simulink model "FourBarCrank_2"  (Simulink 7.0)
settings: Solver=ode1  StartTime=0.0  StopTime=inf  FixedStep=0.001  RelTol=1e-3
libraries: mblibv1 x23
settings Model: Creator=colinlea  LastModifiedBy=colinlea  ExtModeTrigDuration=10000
settings SolverCC: PositivePriorityOrder=on
settings RTWCC: SystemTargetFile=quarc_windows.tlc  TemplateMakefile=quarc_default_tmf  Description=QuaRC Win32 Target  ProcessScript=quarc_windows_make_rtw_hook
settings STFCustomTargetCC: TargetPreCompLibLocation=C:\DOCUME~1\ALLUSE~1\APPLIC~1\QuaRC\lib\2007b\windows\release  GenFloatMathFcnCalls=ANSI_C  SystemTargetFile=quarc_windows.tlc
settings GRTTargetCC: TargetPreCompLibLocation=C:\DOCUME~1\ALLUSE~1\APPLIC~1\QuaRC\lib\2007b\windows\release  CompOptLevelCompliant=off  MatFileLogging=off  ExtMode=on  ExtModeMexFile=quarc_comm
settings SimMechanicsCC: VisOnUpdateDiagram=on  VisDuringSimulation=on

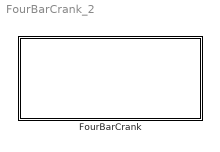
== system FourBarCrank_2 ==
  FourBarCrank : Subsystem

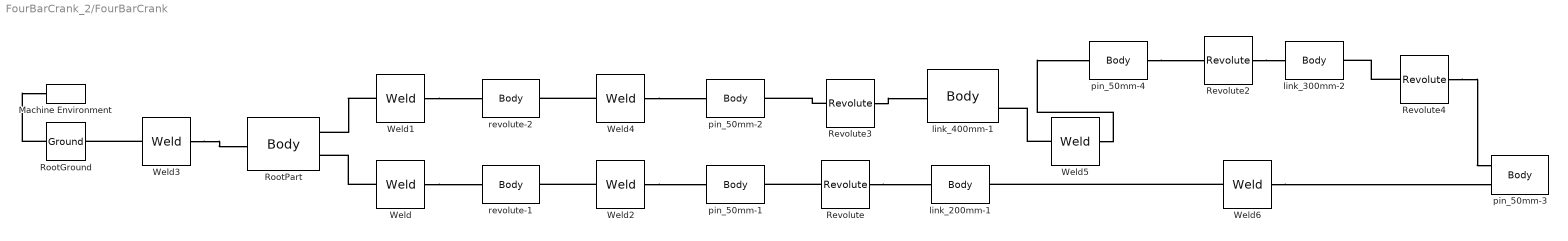
== system FourBarCrank_2/FourBarCrank ==
  Machine Environment : mblibv1/Bodies/Machine Environment  Orientation=left  DialogController=MECH.DialogSource  SystemSampleTime=-1  PortType=env  PhysicalDomain=Mechanical  DialogTemplateClass=MECH.MachineEnvironment  SyncWhenCopied=off  Gravity=[0 -9.81 0]  GravityUnits=m/s^2  GravityAsSignal=off  Dimensionality=Auto-detect  AnalysisType=Forward dynamics  LinearAssemblyTolerance=1e-3  LinearAssemblyToleranceUnits=m  AngularAssemblyTolerance=1e-3  AngularAssemblyToleranceUnits=rad  ConstraintSolverType=Stabilizing  ConstraintRelTolerance=1e-4  ConstraintAbsTolerance=1e-4  UseRobustSingularityHandling=off  RedundancyAnalysisToleranceType=Automatically select tolerance  RedundancyAnalysisTolerance=1e-14  StatePerturbationType=Fixed  PerturbationSize=1e-5  VisualizeMachine=on
  Revolute{,2..4} (4 alike) : mblibv1/Joints/Revolute  DialogController=MECH.DynMechDlgSource  PhysicalDomain=mechanical  SubClassName=Unknown  LeftPortType=blob  RightPortType=blob  LConnTagsString=__newl0  RConnTagsString=__newr0  NumSAPorts=0  CutJoint=off  MarkAsCut=off  Primitives=prismatic  PrimitiveProps=R1$WORLD$[0 0 1]$revolute  DialogClass=JointBlock  R1Axis=[0 0 1]
  RootGround : mblibv1/Bodies/Ground  DialogController=MECH.DynMechDlgSource  SystemSampleTime=-1  LeftPortType=env  RightPortType=workingframe  PhysicalDomain=Mechanical  DialogClass=GroundBlock  CoordPosition=[0.078493 0.18375 0.040178]  CoordPositionUnits=m  StateVectorMgrId=6  MachineId=[6 0]  ShowEnvPort=on
  RootPart : mblibv1/Bodies/Body  DialogController=MECH.DynMechDlgSource  PhysicalDomain=mechanical  SubClassName=Unknown  LeftPortType=workingframe  RightPortType=workingframe  LConnTagsString=CS4  RConnTagsString=CS3|CS2  DialogClass=MechanicalBodyBlock  Mass=0  MassUnits=kg  InertiaUnits=kg*m^2  Inertia=[0 0 0;0 0 0;0 0 0]  ShapeDims=[1 1]  ShapeUnits=m  ShapeUse=false  Density=1  DensityUnits=kg/m^3  DensityUse=false  CG=Right$CG$[0.078493 0.18375 0.040178]$WORLD$WORLD$m$[1 0 0;0 1 0;0 0 1]$3x3 Transform$rad$WORLD$  WorkingFrames=Right$CS3$[0.29621 0.0034984 0.010586]$WORLD$WORLD$m$[1 0 0;0 1 0;0 0 1]$3x3 Transform$rad$WORLD$true#Left$CS4$[0.078493 0.18375 0.040178]$WORLD$WORLD$m$[1 0 0;0 1 0;0 0 1]$3x3 Transform$rad$WORLD$true#Right$CS2$[-0.0037925 0.0034984 0.010586]$WORLD$WORLD$m$[1 0 0;0 1 0;0 0 1]$3x3 Transform$rad$WORLD$true#Right$CS1$[0 0 0]$WORLD$WORLD$m$[1 0 0;0 1 0;0 0 1]$3x3 Transform$rad$WORLD$  CGPos=[0.078493 0.18375 0.040178]  CGRot=[1 0 0;0 1 0;0 0 1]  CS0Pos=[]  CS0Rot=[]  CS1Pos=[0 0 0]  CS1Rot=[1 0 0;0 1 0;0 0 1]  CS2Pos=[-0.0037925 0.0034984 0.010586]  CS2Rot=[1 0 0;0 1 0;0 0 1]  CS3Pos=[0.29621 0.0034984 0.010586]  CS3Rot=[1 0 0;0 1 0;0 0 1]  CS4Pos=[0.078493 0.18375 0.040178]  CS4Rot=[1 0 0;0 1 0;0 0 1]  CS5Pos=[]  CS5Rot=[]  CS6Pos=[]  CS6Rot=[]  CS7Pos=[]  CS7Rot=[]  CS8Pos=[]  CS8Rot=[]  CS9Pos=[]  CS9Rot=[]  CS10Pos=[]  CS10Rot=[]  CS11Pos=[]  CS11Rot=[]  CS12Pos=[]  CS12Rot=[]  CS13Pos=[]  CS13Rot=[]  CS14Pos=[]  CS14Rot=[]  CS15Pos=[]  CS15Rot=[]  CS16Pos=[]  CS16Rot=[]  CS17Pos=[]  CS17Rot=[]  CS18Pos=[]  CS18Rot=[]  CS19Pos=[]  CS19Rot=[]  CS20Pos=[]  CS20Rot=[]
  Weld{,1..6} (7 alike) : mblibv1/Joints/Weld  DialogController=MECH.DynMechDlgSource  PhysicalDomain=mechanical  SubClassName=Unknown  LeftPortType=blob  RightPortType=blob  LConnTagsString=__newl0  RConnTagsString=__newr0  NumSAPorts=0  CutJoint=off  MarkAsCut=off  Primitives=weld  PrimitiveProps=W$WORLD$[0.57735 0.57735 0.57735]$weld  DialogClass=JointBlock  WAxis=[0.57735 0.57735 0.57735]
  link_200mm-1 : mblibv1/Bodies/Body  DialogController=MECH.DynMechDlgSource  PhysicalDomain=mechanical  SubClassName=Unknown  LeftPortType=workingframe  RightPortType=workingframe  LConnTagsString=CS2  RConnTagsString=CS3  DialogClass=MechanicalBodyBlock  Mass=0.091178  MassUnits=kg  InertiaUnits=kg*m^2  Inertia=[8.8204e-006 -2.3562e-008 0;-2.3562e-008 0.00032735 0;0 0 0.00033275]  ShapeDims=[1 1]  ShapeUnits=m  ShapeUse=false  Density=1  DensityUnits=kg/m^3  DensityUse=false  CG=Right$CG$[-0.060969 0.096785 0.048086]$Adjoining$Adjoining$m$[-0.57175 -0.82043 0;0.82043 -0.57175 0;0 0 1]$3x3 Transform$rad$WORLD$false  WorkingFrames=Right$CS3$[0 0 0]$WORLD$WORLD$m$[1 0 0;0 1 0;0 0 1]$3x3 Transform$rad$WORLD$true#Left$CS2$[0 0 0]$WORLD$WORLD$m$[1 0 0;0 1 0;0 0 1]$3x3 Transform$rad$WORLD$true#Right$CS1$[-0.1181 0.17886 0.040586]$WORLD$WORLD$m$[-0.57175 -0.82043 0;0.82043 -0.57175 0;0 0 1]$3x3 Transform$rad$WORLD$false  CGPos=[-0.060969 0.096785 0.048086]  CGRot=[-0.57175 -0.82043 0;0.82043 -0.57175 0;0 0 1]  CS0Pos=[]  CS0Rot=[]  CS1Pos=[-0.1181 0.17886 0.040586]  CS1Rot=[-0.57175 -0.82043 0;0.82043 -0.57175 0;0 0 1]  CS2Pos=[0 0 0]  CS2Rot=[1 0 0;0 1 0;0 0 1]  CS3Pos=[0 0 0]  CS3Rot=[1 0 0;0 1 0;0 0 1]  CS4Pos=[]  CS4Rot=[]  CS5Pos=[]  CS5Rot=[]  CS6Pos=[]  CS6Rot=[]  CS7Pos=[]  CS7Rot=[]  CS8Pos=[]  CS8Rot=[]  CS9Pos=[]  CS9Rot=[]  CS10Pos=[]  CS10Rot=[]  CS11Pos=[]  CS11Rot=[]  CS12Pos=[]  CS12Rot=[]  CS13Pos=[]  CS13Rot=[]  CS14Pos=[]  CS14Rot=[]  CS15Pos=[]  CS15Rot=[]  CS16Pos=[]  CS16Rot=[]  CS17Pos=[]  CS17Rot=[]  CS18Pos=[]  CS18Rot=[]  CS19Pos=[]  CS19Rot=[]  CS20Pos=[]  CS20Rot=[]
  link_300mm-2 : mblibv1/Bodies/Body  DialogController=MECH.DynMechDlgSource  PhysicalDomain=mechanical  SubClassName=Unknown  LeftPortType=workingframe  RightPortType=workingframe  LConnTagsString=CS2  RConnTagsString=CS3  DialogClass=MechanicalBodyBlock  Mass=0.13618  MassUnits=kg  InertiaUnits=kg*m^2  Inertia=[1.3039e-005 0 0;0 0.0010622 0;0 0 0.0010701]  ShapeDims=[1 1]  ShapeUnits=m  ShapeUse=false  Density=1  DensityUnits=kg/m^3  DensityUse=false  CG=Right$CG$[-0.0026001 0.27456 0.033086]$Adjoining$Adjoining$m$[0.77001 -0.63804 0;0.63804 0.77001 0;0 0 1]$3x3 Transform$rad$WORLD$false  WorkingFrames=Left$CS2$[0.1129 0.37027 0.0055863]$WORLD$WORLD$m$[1 0 0;0 1 0;0 0 1]$3x3 Transform$rad$WORLD$true#Right$CS3$[-0.1181 0.17886 0.040586]$WORLD$WORLD$m$[1 0 0;0 1 0;0 0 1]$3x3 Transform$rad$WORLD$true#Right$CS1$[0.1129 0.37027 0.025586]$WORLD$WORLD$m$[0.77001 -0.63804 0;0.63804 0.77001 0;0 0 1]$3x3 Transform$rad$WORLD$false  CGPos=[-0.0026001 0.27456 0.033086]  CGRot=[0.77001 -0.63804 0;0.63804 0.77001 0;0 0 1]  CS0Pos=[]  CS0Rot=[]  CS1Pos=[0.1129 0.37027 0.025586]  CS1Rot=[0.77001 -0.63804 0;0.63804 0.77001 0;0 0 1]  CS2Pos=[0.1129 0.37027 0.0055863]  CS2Rot=[1 0 0;0 1 0;0 0 1]  CS3Pos=[-0.1181 0.17886 0.040586]  CS3Rot=[1 0 0;0 1 0;0 0 1]  CS4Pos=[]  CS4Rot=[]  CS5Pos=[]  CS5Rot=[]  CS6Pos=[]  CS6Rot=[]  CS7Pos=[]  CS7Rot=[]  CS8Pos=[]  CS8Rot=[]  CS9Pos=[]  CS9Rot=[]  CS10Pos=[]  CS10Rot=[]  CS11Pos=[]  CS11Rot=[]  CS12Pos=[]  CS12Rot=[]  CS13Pos=[]  CS13Rot=[]  CS14Pos=[]  CS14Rot=[]  CS15Pos=[]  CS15Rot=[]  CS16Pos=[]  CS16Rot=[]  CS17Pos=[]  CS17Rot=[]  CS18Pos=[]  CS18Rot=[]  CS19Pos=[]  CS19Rot=[]  CS20Pos=[]  CS20Rot=[]
  link_400mm-1 : mblibv1/Bodies/Body  DialogController=MECH.DynMechDlgSource  PhysicalDomain=mechanical  SubClassName=Unknown  LeftPortType=workingframe  RightPortType=workingframe  LConnTagsString=CS3  RConnTagsString=CS4|CS2  DialogClass=MechanicalBodyBlock  Mass=0.18118  MassUnits=kg  InertiaUnits=kg*m^2  Inertia=[1.7258e-005 0 0;0 0.0024779 0;0 0 0.0024883]  ShapeDims=[1 1]  ShapeUnits=m  ShapeUse=false  Density=1  DensityUnits=kg/m^3  DensityUse=false  CG=Right$CG$[0.20455 0.19251 0.048086]$Adjoining$Adjoining$m$[0.45827 0.88882 0;-0.88882 0.45827 0;0 0 1]$3x3 Transform$rad$WORLD$false  WorkingFrames=Right$CS4$[0 0 0]$WORLD$WORLD$m$[1 0 0;0 1 0;0 0 1]$3x3 Transform$rad$WORLD$true#Left$CS3$[0 0 0]$WORLD$WORLD$m$[1 0 0;0 1 0;0 0 1]$3x3 Transform$rad$WORLD$true#Right$CS2$[0 0 0]$WORLD$WORLD$m$[1 0 0;0 1 0;0 0 1]$3x3 Transform$rad$WORLD$true#Right$CS1$[0.29621 0.014744 0.040586]$WORLD$WORLD$m$[0.45827 0.88882 0;-0.88882 0.45827 0;0 0 1]$3x3 Transform$rad$WORLD$false  CGPos=[0.20455 0.19251 0.048086]  CGRot=[0.45827 0.88882 0;-0.88882 0.45827 0;0 0 1]  CS0Pos=[]  CS0Rot=[]  CS1Pos=[0.29621 0.014744 0.040586]  CS1Rot=[0.45827 0.88882 0;-0.88882 0.45827 0;0 0 1]  CS2Pos=[0 0 0]  CS2Rot=[1 0 0;0 1 0;0 0 1]  CS3Pos=[0 0 0]  CS3Rot=[1 0 0;0 1 0;0 0 1]  CS4Pos=[0 0 0]  CS4Rot=[1 0 0;0 1 0;0 0 1]  CS5Pos=[]  CS5Rot=[]  CS6Pos=[]  CS6Rot=[]  CS7Pos=[]  CS7Rot=[]  CS8Pos=[]  CS8Rot=[]  CS9Pos=[]  CS9Rot=[]  CS10Pos=[]  CS10Rot=[]  CS11Pos=[]  CS11Rot=[]  CS12Pos=[]  CS12Rot=[]  CS13Pos=[]  CS13Rot=[]  CS14Pos=[]  CS14Rot=[]  CS15Pos=[]  CS15Rot=[]  CS16Pos=[]  CS16Rot=[]  CS17Pos=[]  CS17Rot=[]  CS18Pos=[]  CS18Rot=[]  CS19Pos=[]  CS19Rot=[]  CS20Pos=[]  CS20Rot=[]
  pin_50mm-1 : mblibv1/Bodies/Body  DialogController=MECH.DynMechDlgSource  PhysicalDomain=mechanical  SubClassName=Unknown  LeftPortType=workingframe  RightPortType=workingframe  LConnTagsString=CS3  RConnTagsString=CS2  DialogClass=MechanicalBodyBlock  Mass=0.015708  MassUnits=kg  InertiaUnits=kg*m^2  Inertia=[3.6652e-006 0 0;0 3.6652e-006 0;0 0 7.854e-007]  ShapeDims=[1 1]  ShapeUnits=m  ShapeUse=false  Density=1  DensityUnits=kg/m^3  DensityUse=false  CG=Right$CG$[-0.0037925 0.014744 0.030586]$WORLD$WORLD$m$[1 0 0;0 1 0;0 0 1]$3x3 Transform$rad$WORLD$  WorkingFrames=Right$CS2$[0 0 0]$WORLD$WORLD$m$[1 0 0;0 1 0;0 0 1]$3x3 Transform$rad$WORLD$true#Left$CS3$[-0.0037925 0.014744 0.015586]$WORLD$WORLD$m$[1 0 0;0 1 0;0 0 1]$3x3 Transform$rad$WORLD$true#Right$CS1$[-0.0037925 0.014744 0.0055863]$WORLD$WORLD$m$[1 0 0;0 1 0;0 0 1]$3x3 Transform$rad$WORLD$  CGPos=[-0.0037925 0.014744 0.030586]  CGRot=[1 0 0;0 1 0;0 0 1]  CS0Pos=[]  CS0Rot=[]  CS1Pos=[-0.0037925 0.014744 0.0055863]  CS1Rot=[1 0 0;0 1 0;0 0 1]  CS2Pos=[0 0 0]  CS2Rot=[1 0 0;0 1 0;0 0 1]  CS3Pos=[-0.0037925 0.014744 0.015586]  CS3Rot=[1 0 0;0 1 0;0 0 1]  CS4Pos=[]  CS4Rot=[]  CS5Pos=[]  CS5Rot=[]  CS6Pos=[]  CS6Rot=[]  CS7Pos=[]  CS7Rot=[]  CS8Pos=[]  CS8Rot=[]  CS9Pos=[]  CS9Rot=[]  CS10Pos=[]  CS10Rot=[]  CS11Pos=[]  CS11Rot=[]  CS12Pos=[]  CS12Rot=[]  CS13Pos=[]  CS13Rot=[]  CS14Pos=[]  CS14Rot=[]  CS15Pos=[]  CS15Rot=[]  CS16Pos=[]  CS16Rot=[]  CS17Pos=[]  CS17Rot=[]  CS18Pos=[]  CS18Rot=[]  CS19Pos=[]  CS19Rot=[]  CS20Pos=[]  CS20Rot=[]
  pin_50mm-2 : mblibv1/Bodies/Body  DialogController=MECH.DynMechDlgSource  PhysicalDomain=mechanical  SubClassName=Unknown  LeftPortType=workingframe  RightPortType=workingframe  LConnTagsString=CS3  RConnTagsString=CS2  DialogClass=MechanicalBodyBlock  Mass=0.015708  MassUnits=kg  InertiaUnits=kg*m^2  Inertia=[3.6652e-006 0 0;0 3.6652e-006 0;0 0 7.854e-007]  ShapeDims=[1 1]  ShapeUnits=m  ShapeUse=false  Density=1  DensityUnits=kg/m^3  DensityUse=false  CG=Right$CG$[0.29621 0.014744 0.030586]$WORLD$WORLD$m$[1 0 0;0 1 0;0 0 1]$3x3 Transform$rad$WORLD$  WorkingFrames=Right$CS2$[0 0 0]$WORLD$WORLD$m$[1 0 0;0 1 0;0 0 1]$3x3 Transform$rad$WORLD$true#Left$CS3$[0 0 0]$WORLD$WORLD$m$[1 0 0;0 1 0;0 0 1]$3x3 Transform$rad$WORLD$true#Right$CS1$[0.29621 0.014744 0.0055863]$WORLD$WORLD$m$[1 0 0;0 1 0;0 0 1]$3x3 Transform$rad$WORLD$  CGPos=[0.29621 0.014744 0.030586]  CGRot=[1 0 0;0 1 0;0 0 1]  CS0Pos=[]  CS0Rot=[]  CS1Pos=[0.29621 0.014744 0.0055863]  CS1Rot=[1 0 0;0 1 0;0 0 1]  CS2Pos=[0 0 0]  CS2Rot=[1 0 0;0 1 0;0 0 1]  CS3Pos=[0 0 0]  CS3Rot=[1 0 0;0 1 0;0 0 1]  CS4Pos=[]  CS4Rot=[]  CS5Pos=[]  CS5Rot=[]  CS6Pos=[]  CS6Rot=[]  CS7Pos=[]  CS7Rot=[]  CS8Pos=[]  CS8Rot=[]  CS9Pos=[]  CS9Rot=[]  CS10Pos=[]  CS10Rot=[]  CS11Pos=[]  CS11Rot=[]  CS12Pos=[]  CS12Rot=[]  CS13Pos=[]  CS13Rot=[]  CS14Pos=[]  CS14Rot=[]  CS15Pos=[]  CS15Rot=[]  CS16Pos=[]  CS16Rot=[]  CS17Pos=[]  CS17Rot=[]  CS18Pos=[]  CS18Rot=[]  CS19Pos=[]  CS19Rot=[]  CS20Pos=[]  CS20Rot=[]
  pin_50mm-3 : mblibv1/Bodies/Body  DialogController=MECH.DynMechDlgSource  PhysicalDomain=mechanical  SubClassName=Unknown  LeftPortType=workingframe  RightPortType=workingframe  LConnTagsString=CS3|CS2  DialogClass=MechanicalBodyBlock  Mass=0.015708  MassUnits=kg  InertiaUnits=kg*m^2  Inertia=[3.6652e-006 0 0;0 3.6652e-006 0;0 0 7.854e-007]  ShapeDims=[1 1]  ShapeUnits=m  ShapeUse=false  Density=1  DensityUnits=kg/m^3  DensityUse=false  CG=Right$CG$[-0.1181 0.17886 0.030586]$WORLD$WORLD$m$[1 0 0;0 1 0;0 0 1]$3x3 Transform$rad$WORLD$  WorkingFrames=Left$CS3$[-0.1181 0.17886 0.040586]$WORLD$WORLD$m$[1 0 0;0 1 0;0 0 1]$3x3 Transform$rad$WORLD$true#Left$CS2$[0 0 0]$WORLD$WORLD$m$[1 0 0;0 1 0;0 0 1]$3x3 Transform$rad$WORLD$true#Right$CS1$[-0.1181 0.17886 0.0055863]$WORLD$WORLD$m$[1 0 0;0 1 0;0 0 1]$3x3 Transform$rad$WORLD$  CGPos=[-0.1181 0.17886 0.030586]  CGRot=[1 0 0;0 1 0;0 0 1]  CS0Pos=[]  CS0Rot=[]  CS1Pos=[-0.1181 0.17886 0.0055863]  CS1Rot=[1 0 0;0 1 0;0 0 1]  CS2Pos=[0 0 0]  CS2Rot=[1 0 0;0 1 0;0 0 1]  CS3Pos=[-0.1181 0.17886 0.040586]  CS3Rot=[1 0 0;0 1 0;0 0 1]  CS4Pos=[]  CS4Rot=[]  CS5Pos=[]  CS5Rot=[]  CS6Pos=[]  CS6Rot=[]  CS7Pos=[]  CS7Rot=[]  CS8Pos=[]  CS8Rot=[]  CS9Pos=[]  CS9Rot=[]  CS10Pos=[]  CS10Rot=[]  CS11Pos=[]  CS11Rot=[]  CS12Pos=[]  CS12Rot=[]  CS13Pos=[]  CS13Rot=[]  CS14Pos=[]  CS14Rot=[]  CS15Pos=[]  CS15Rot=[]  CS16Pos=[]  CS16Rot=[]  CS17Pos=[]  CS17Rot=[]  CS18Pos=[]  CS18Rot=[]  CS19Pos=[]  CS19Rot=[]  CS20Pos=[]  CS20Rot=[]
  pin_50mm-4 : mblibv1/Bodies/Body  DialogController=MECH.DynMechDlgSource  PhysicalDomain=mechanical  SubClassName=Unknown  LeftPortType=workingframe  RightPortType=workingframe  LConnTagsString=CS2  RConnTagsString=CS1  DialogClass=MechanicalBodyBlock  Mass=0.015708  MassUnits=kg  InertiaUnits=kg*m^2  Inertia=[3.6652e-006 0 0;0 3.6652e-006 0;0 0 7.854e-007]  ShapeDims=[1 1]  ShapeUnits=m  ShapeUse=false  Density=1  DensityUnits=kg/m^3  DensityUse=false  CG=Right$CG$[0.1129 0.37027 0.030586]$WORLD$WORLD$m$[1 0 0;0 1 0;0 0 1]$3x3 Transform$rad$WORLD$false  WorkingFrames=Left$CS2$[0 0 0]$WORLD$WORLD$m$[1 0 0;0 1 0;0 0 1]$3x3 Transform$rad$WORLD$true#Right$CS1$[0.1129 0.37027 0.0055863]$WORLD$WORLD$m$[1 0 0;0 1 0;0 0 1]$3x3 Transform$rad$WORLD$true  CGPos=[0.1129 0.37027 0.030586]  CGRot=[1 0 0;0 1 0;0 0 1]  CS0Pos=[]  CS0Rot=[]  CS1Pos=[0.1129 0.37027 0.0055863]  CS1Rot=[1 0 0;0 1 0;0 0 1]  CS2Pos=[0 0 0]  CS2Rot=[1 0 0;0 1 0;0 0 1]  CS3Pos=[]  CS3Rot=[]  CS4Pos=[]  CS4Rot=[]  CS5Pos=[]  CS5Rot=[]  CS6Pos=[]  CS6Rot=[]  CS7Pos=[]  CS7Rot=[]  CS8Pos=[]  CS8Rot=[]  CS9Pos=[]  CS9Rot=[]  CS10Pos=[]  CS10Rot=[]  CS11Pos=[]  CS11Rot=[]  CS12Pos=[]  CS12Rot=[]  CS13Pos=[]  CS13Rot=[]  CS14Pos=[]  CS14Rot=[]  CS15Pos=[]  CS15Rot=[]  CS16Pos=[]  CS16Rot=[]  CS17Pos=[]  CS17Rot=[]  CS18Pos=[]  CS18Rot=[]  CS19Pos=[]  CS19Rot=[]  CS20Pos=[]  CS20Rot=[]
  revolute-1 : mblibv1/Bodies/Body  DialogController=MECH.DynMechDlgSource  PhysicalDomain=mechanical  SubClassName=Unknown  LeftPortType=workingframe  RightPortType=workingframe  LConnTagsString=CS2  RConnTagsString=CS3  DialogClass=MechanicalBodyBlock  Mass=0.0098927  MassUnits=kg  InertiaUnits=kg*m^2  Inertia=[1.3308e-006 0 0;0 1.5819e-006 0;0 0 2.7478e-006]  ShapeDims=[1 1]  ShapeUnits=m  ShapeUse=false  Density=1  DensityUnits=kg/m^3  DensityUse=false  CG=Right$CG$[-0.0037925 0.0034984 0.010586]$WORLD$WORLD$m$[1 0 0;0 1 0;0 0 1]$3x3 Transform$rad$WORLD$  WorkingFrames=Left$CS2$[-0.0037925 0.0034984 0.010586]$WORLD$WORLD$m$[1 0 0;0 1 0;0 0 1]$3x3 Transform$rad$WORLD$true#Right$CS3$[-0.0037925 0.014744 0.015586]$WORLD$WORLD$m$[1 0 0;0 1 0;0 0 1]$3x3 Transform$rad$WORLD$true#Right$CS1$[-0.0039028 -0.0051912 0.0055863]$WORLD$WORLD$m$[1 0 0;0 1 0;0 0 1]$3x3 Transform$rad$WORLD$  CGPos=[-0.0037925 0.0034984 0.010586]  CGRot=[1 0 0;0 1 0;0 0 1]  CS0Pos=[]  CS0Rot=[]  CS1Pos=[-0.0039028 -0.0051912 0.0055863]  CS1Rot=[1 0 0;0 1 0;0 0 1]  CS2Pos=[-0.0037925 0.0034984 0.010586]  CS2Rot=[1 0 0;0 1 0;0 0 1]  CS3Pos=[-0.0037925 0.014744 0.015586]  CS3Rot=[1 0 0;0 1 0;0 0 1]  CS4Pos=[]  CS4Rot=[]  CS5Pos=[]  CS5Rot=[]  CS6Pos=[]  CS6Rot=[]  CS7Pos=[]  CS7Rot=[]  CS8Pos=[]  CS8Rot=[]  CS9Pos=[]  CS9Rot=[]  CS10Pos=[]  CS10Rot=[]  CS11Pos=[]  CS11Rot=[]  CS12Pos=[]  CS12Rot=[]  CS13Pos=[]  CS13Rot=[]  CS14Pos=[]  CS14Rot=[]  CS15Pos=[]  CS15Rot=[]  CS16Pos=[]  CS16Rot=[]  CS17Pos=[]  CS17Rot=[]  CS18Pos=[]  CS18Rot=[]  CS19Pos=[]  CS19Rot=[]  CS20Pos=[]  CS20Rot=[]
  revolute-2 : mblibv1/Bodies/Body  DialogController=MECH.DynMechDlgSource  PhysicalDomain=mechanical  SubClassName=Unknown  LeftPortType=workingframe  RightPortType=workingframe  LConnTagsString=CS2  RConnTagsString=CS3  DialogClass=MechanicalBodyBlock  Mass=0.0098927  MassUnits=kg  InertiaUnits=kg*m^2  Inertia=[1.3308e-006 0 0;0 1.5819e-006 0;0 0 2.7478e-006]  ShapeDims=[1 1]  ShapeUnits=m  ShapeUse=false  Density=1  DensityUnits=kg/m^3  DensityUse=false  CG=Right$CG$[0.29621 0.0034984 0.010586]$WORLD$WORLD$m$[1 0 0;0 1 0;0 0 1]$3x3 Transform$rad$WORLD$  WorkingFrames=Left$CS2$[0.29621 0.0034984 0.010586]$WORLD$WORLD$m$[1 0 0;0 1 0;0 0 1]$3x3 Transform$rad$WORLD$true#Right$CS3$[0 0 0]$WORLD$WORLD$m$[1 0 0;0 1 0;0 0 1]$3x3 Transform$rad$WORLD$true#Right$CS1$[0.2961 -0.0051912 0.0055863]$WORLD$WORLD$m$[1 0 0;0 1 0;0 0 1]$3x3 Transform$rad$WORLD$  CGPos=[0.29621 0.0034984 0.010586]  CGRot=[1 0 0;0 1 0;0 0 1]  CS0Pos=[]  CS0Rot=[]  CS1Pos=[0.2961 -0.0051912 0.0055863]  CS1Rot=[1 0 0;0 1 0;0 0 1]  CS2Pos=[0.29621 0.0034984 0.010586]  CS2Rot=[1 0 0;0 1 0;0 0 1]  CS3Pos=[0 0 0]  CS3Rot=[1 0 0;0 1 0;0 0 1]  CS4Pos=[]  CS4Rot=[]  CS5Pos=[]  CS5Rot=[]  CS6Pos=[]  CS6Rot=[]  CS7Pos=[]  CS7Rot=[]  CS8Pos=[]  CS8Rot=[]  CS9Pos=[]  CS9Rot=[]  CS10Pos=[]  CS10Rot=[]  CS11Pos=[]  CS11Rot=[]  CS12Pos=[]  CS12Rot=[]  CS13Pos=[]  CS13Rot=[]  CS14Pos=[]  CS14Rot=[]  CS15Pos=[]  CS15Rot=[]  CS16Pos=[]  CS16Rot=[]  CS17Pos=[]  CS17Rot=[]  CS18Pos=[]  CS18Rot=[]  CS19Pos=[]  CS19Rot=[]  CS20Pos=[]  CS20Rot=[]
  connections:
  Weld/LConn1 -- RootPart/RConn2
  Weld/RConn1 -- revolute-1/LConn1
  Weld1/LConn1 -- RootPart/RConn1
  Weld1/RConn1 -- revolute-2/LConn1
  Revolute/LConn1 -- pin_50mm-1/RConn1
  Revolute/RConn1 -- link_200mm-1/LConn1
  Weld6/LConn1 -- link_200mm-1/RConn1
  Weld6/RConn1 -- pin_50mm-3/LConn2
  Weld5/LConn1 -- link_400mm-1/RConn2
  Weld5/RConn1 -- pin_50mm-4/LConn1
  Revolute3/LConn1 -- pin_50mm-2/RConn1
  Revolute3/RConn1 -- link_400mm-1/LConn1
  Weld2/LConn1 -- revolute-1/RConn1
  Weld2/RConn1 -- pin_50mm-1/LConn1
  Weld4/LConn1 -- revolute-2/RConn1
  Weld4/RConn1 -- pin_50mm-2/LConn1
  Revolute4/LConn1 -- link_300mm-2/RConn1
  Revolute4/RConn1 -- pin_50mm-3/LConn1
  Weld3/LConn1 -- RootGround/RConn1
  Weld3/RConn1 -- RootPart/LConn1
  RootGround/LConn1 -- Machine Environment/RConn1
  pin_50mm-4/RConn1 -- Revolute2/LConn1
  Revolute2/RConn1 -- link_300mm-2/LConn1
